simulink subsystem "VSNoiseModel"  (R2020b)
settings: Solver=VariableStepAuto  StartTime=0.0  StopTime=10.0  RelTol=1e-3
model mask{noise_perc=0, noise_sample_time=-1}
settings Model: Creator=marco  LastModifiedBy=marco

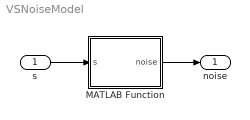
== system VSNoiseModel ==
  s : Inport
  MATLAB Function : MATLAB Function  TreatAsAtomicUnit=on  SystemSampleTime=noise_sample_time
  noise : Outport
  wires:
  s/1 -> MATLAB Function/1(s)
  MATLAB Function/1(noise) -> noise/1

== matlab function VSNoiseModel/MATLAB Function ==
  data: s input; noise output; noise_perc parameter
function noise = fcn(s,noise_perc)

N = numel(s)/3;

s_ = reshape(s,3,N);
noise_ = zeros(size(s_));

a = -1; b = 1;
for i=1:N
    r_ = a + (b-a).*rand(3,1);
    noise_(:,i) = r_ * s_(3,i) * noise_perc;
end

noise = noise_(:);
